simulink model "rtwdemo_cscpredef"  (Simulink 6.0)
settings: Solver=FixedStepDiscrete  StartTime=0.0  StopTime=10.0  FixedStep=1.0  RelTol=1e-3
PostLoadFcn:
  | rtwdemo_cscpredef_data;
undefined symbols (not defined in the file or in its folder): O2limit, pressurelimit, rpmlimit, templimit
libraries: rtwdemowidgets x2
settings Model: CovMetricSettings=d  Creator=The MathWorks Inc.  LastModifiedBy=batserve  ExtModeAutoUpdateStatusClock=off
settings DataIOCC: SaveOutput=off  SaveTime=off  SignalLoggingName=sigsOut
settings OptimizationCC: InlineParams=on  EnforceIntegerDowncast=off  StateBitsets=on  DataBitsets=on  UseTempVars=on  ZeroExternalMemoryAtStartup=off  ZeroInternalMemoryAtStartup=off  InitFltsAndDblsToZero=off  NoFixptDivByZeroProtection=on  OptimizeModelRefInitCode=on  LifeSpan=1
settings DebuggingCC: CheckExecutionContextPreStartOutputMsg=on  CheckExecutionContextRuntimeOutputMsg=on  SignalResolutionControl=TryResolveAll  SolverPrmCheckMsg=none
settings HardwareCC: TargetHWDeviceType=32-bit Generic
settings RTWCC: SystemTargetFile=ert.tlc  TLCOptions=-p0 -aWarnNonSaturatedBlocks=0  GenCodeOnly=on  TemplateMakefile=ert_default_tmf  GenerateReport=on  RTWVerbose=off  ProcessScript=ert_make_rtw_hook  IncludeHyperlinkInReport=on  LaunchReport=on
settings CodeAppCC: ForceParamTrailComments=on  IgnoreCustomStorageClasses=off  SimulinkDataObjDesc=on  PrefixModelToSubsysFcnNames=off  CustomSymbolStr=$N$M  InsertBlockDesc=on
settings ERTTargetCC: TargetFcnLib=ansi_tfl_tmw.mat  GenFloatMathFcnCalls=ANSI_C  GenerateSampleERTMain=on  IncludeMdlTerminateFcn=off  SupportNonFinite=off  SupportContinuousTime=on  SupportNonInlinedSFcns=on  InlinedParameterPlacement=NonHierarchical  RootIOFormat=Individual Arguments  ERTCustomFileTemplate=example_file_process.tlc  InitialValueSource=Model

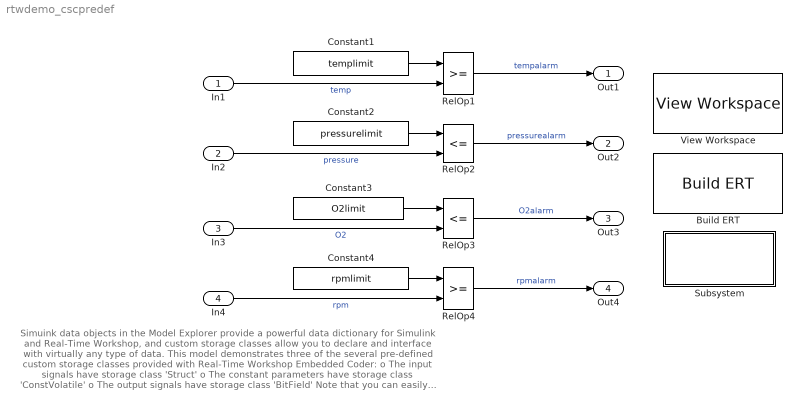
== system rtwdemo_cscpredef ==
  note: Simuink data objects in the Model Explorer provide a powerful data dictionary for Simulink
      | and Real-Time Workshop, and custom storage classes allow you to declare and interface with
      | virtually any type of data.  This model demonstrates three of the several pre-defined
      | custom storage classes provided with Real-Time Workshop Embedded Coder:
      |
      | o The input signals have storage class 'Struct'
      | o The constant parameters have storage class 'ConstVolatile'
      | o The output signals have storage class 'BitField'
      |
      | Note that you can easily create your own custom classes using the Custom Storage Class
      | Designer (type cscdesigner at the MATLAB command line).
  In1 : Inport  Port=1  LatchInput=off
  In2 : Inport  Port=2  LatchInput=off
  In3 : Inport  Port=3  LatchInput=off
  In4 : Inport  Port=4  LatchInput=off
  Build ERT : rtwdemowidgets/Build ERT  attrib_overrides={}
  Constant1 : Constant  Value=templimit
  Constant2 : Constant  Value=pressurelimit
  Constant3 : Constant  Value=O2limit
  Constant4 : Constant  Value=rpmlimit
  RelOp1 : RelationalOperator  InputSameDT=on
  RelOp2 : RelationalOperator  Operator=<=  InputSameDT=on
  RelOp3 : RelationalOperator  Operator=<=  InputSameDT=on
  RelOp4 : RelationalOperator  InputSameDT=on
  Subsystem : Subsystem  PropExecContextAcrossSSBoundary=on
      mask Display: text(.05,.5,['License\nRequirements ..','.'])
  View Workspace : rtwdemowidgets/View Workspace
  Out1 : Outport
  Out2 : Outport  Port=2
  Out3 : Outport  Port=3
  Out4 : Outport  Port=4
  wires:
  In1/1 -> RelOp1/2  "temp"
  RelOp1/1 -> Out1/1  "tempalarm"
  In2/1 -> RelOp2/2  "pressure"
  RelOp2/1 -> Out2/1  "pressurealarm"
  In3/1 -> RelOp3/2  "O2"
  RelOp3/1 -> Out3/1  "O2alarm"
  In4/1 -> RelOp4/2  "rpm"
  RelOp4/1 -> Out4/1  "rpmalarm"
  Constant1/1 -> RelOp1/1
  Constant2/1 -> RelOp2/1
  Constant3/1 -> RelOp3/1
  Constant4/1 -> RelOp4/1

== system rtwdemo_cscpredef/Subsystem ==
  note: You can define, create, and simulate models with Custom Storage Classes with a Simulink license.  However,
      | for the properties to take effect in the generated code, a Real-Time Workshop Embedded Coder license is
      | required.  When generating code for models without an Embedded Coder license the properties are
      | ignored (i.e., the custom storage class value defaults to auto storage.)  In other words, Custom Storage
      | Classes are ignored for GRT targets.
